simulink model "controller"  (R2016a)
settings: Solver=VariableStepAuto  StartTime=0.0  StopTime=10.0  RelTol=1e-3
values from neighbouring files (symbols this model uses):
  A = [-5.1193e-08 -0.0535; -1.8571 -1.2236]    [Controller_Initial_response.m]    (also in Observer_Initial_response.m; System_behaviour_Stability_Controllability_Observability.m)
  B = [-0.227147; 0.324495]    [Controller_Initial_response.m]    (also in Observer_Initial_response.m; System_behaviour_Stability_Controllability_Observability.m)
  C = [1 0]    [Controller_Initial_response.m]    (also in Observer_Initial_response.m; System_behaviour_Stability_Controllability_Observability.m)
  k = 2    [System_behaviour_Stability_Controllability_Observability.m]
settings Model: Creator=User  LastModifiedBy=User

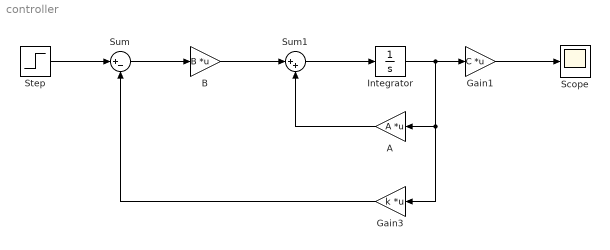
== system controller ==
  A : Gain  Gain=A  Multiplication=Matrix(K*u)
  B : Gain  Gain=B  Multiplication=Matrix(K*u)
  Gain1 : Gain  Gain=C  Multiplication=Matrix(K*u)
  Gain3 : Gain  Gain=k  Multiplication=Matrix(K*u)
  Integrator : Integrator
  Scope : Scope
  Step : Step  After=1.3  SampleTime=0
  Sum : Sum  Inputs=|+-
  Sum1 : Sum  Inputs=|++
  wires:
  Step/1 -> Sum/1
  Sum/1 -> B/1
  B/1 -> Sum1/1
  Sum1/1 -> Integrator/1
  Integrator/1 -> Gain3/1, A/1, Gain1/1
  Gain1/1 -> Scope/1
  A/1 -> Sum1/2
  Gain3/1 -> Sum/2
